simulink library "UndergraduateResearch"  (Simulink 8.1)
settings: Solver=ode45  StartTime=0.0  StopTime=10.0  RelTol=1e-3
undefined symbols (not defined in the file or in its folder): datafiI, datafiQ, i, magnitude
libraries: commchan3 x40, UndergraduateResearch x35, dspxfrm3 x6, dspstat3 x4, dspmtrx3 x4, commseqgen2 x4, dspindex x2, simulink x2, dspbuff3 x1
(part 1 of 2)
settings Model: Creator=dmiralles  LastModifiedBy=dmiralles

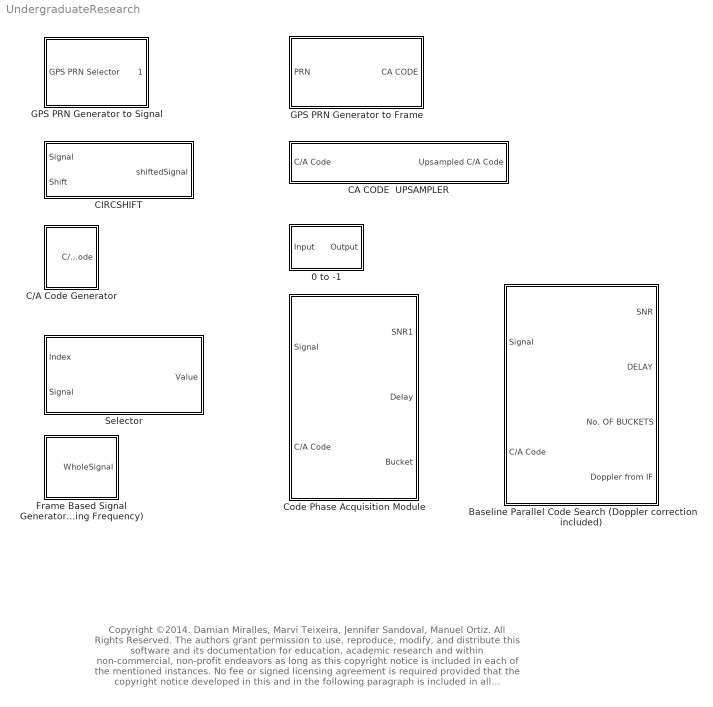
== system UndergraduateResearch ==
  note: Copyright ©2014.  Damian Miralles, Marvi Teixeira, Jennifer Sandoval, Manuel Ortiz. All Rights Reserved.
      | The authors grant permission to use, reproduce, modify, and distribute this software and its documentation for
      | education,  academic research and within non-commercial, non-profit endeavors as long as this copyright notice
      |  is included in each of the mentioned instances. No fee or signed licensing agreement is required provided that
      | the copyright notice developed in this and in the following  paragraph is included in all reproductions,  alterations,
      | and distributions of the software or its  documentation. Contact the authors regarding any commercial licensing needs.
      |
      | THIS EXPERIMENTAL SOFTWARE AND RELATED DOCUMENTATION ARE PROVIDED “AS IS” AND
      |  NO, EXPLICIT OR IMPLICT, CLAIMS REGARDING THEIR ACCURACY OR SUITABILITY ARE MADE.
      | USERS ARE RESPONSIBLE FOR SOFTWARE VALIDATION REGARDING THEIR PARTICULAR
      |  APPLICATION. NO UPDATES WILL BE OFFERED. VERY LIMITED SUPPORT COULD BE PROVIDED,
      |  BUT NOT GUARANTEED, ON A CASE BY CASE BASIS, DEPENDING ON THE AVAILABLE TIME
      |  RESOURCES AT THE TIME OF THE REQUEST.
      | (dmiralles2009@gmail.com,  cc: mteixeir@ieee.org )
  " 0 to -1" : Subsystem  mask(Change 0 to -1){}
      mask help: The blocks performs the conversion of the 0 values to -1. This is used to represent the series as in the polar non-return-to-zero notation which is more easy to handle to perform data analysis.
      mask Help:
      | After code generation, the codes are combined with the navigation data through modulo-2 adders. The exclusive OR operation is used on binary sequences represented by 0’s and 1’s, and its properties are shown in  Table 1.
      | <br>
      | 
      | <table>
      |   <caption>Table 1:Output of the exclusive OR operation</caption>
      |   <tr>
      |     <th>Input</th>
      |     <th>Input</th>
      |     <th>Output</th>
      |   </tr>
      |   <tr>
      |     <td>0</td>
      |     <td>0</td>
      |     <td>0</td>
      |   </tr>
      |   <tr>
      |     <td>0</td>
      |     <td>1</td>
      |     <td>1</td>
      |   </tr>
      |   <tr>
      |     <td>1</td>
      |     <td>0</td>
      |     <td>1</td>
      |   </tr>
      |   <tr>
      |     <td>1</td>
      |     <td>1</td>
      |     <td>0</td>
      |   </tr>
      | </table>
      | 
      | If the binary sequences were represented by the polar non-return-to-zero representation, i.e., 1’s and −1’s, ordinary multiplication could be used instead. The corresponding properties of the multiplication with two binary non-return-to-zero  sequences are shown in Table 2.
      | 
      | <table>
      |   <caption>Table 1:Output of the exclusive OR operation</caption>
      |   <colgroup span="4" class="columns"></colgroup>
      |   <tr>
      |     <th>Input</th>
      |     <th>Input</th>
      |     <th>Output</th>
      |   </tr>
      |   <tr>
      |     <td>-1</td>
      |     <td>-1</td>
      |     <td>1</td>
      |   </tr>
      |   <tr>
      |     <td>-1</td>
      |     <td>1</td>
      |     <td>-1</td>
      |   </tr>
      |   <tr>
      |     <td>1</td>
      |     <td>-1</td>
      |     <td>-1</td>
      |   </tr>
      |   <tr>
      |     <td>1</td>
      |     <td>1</td>
      |     <td>1</td>
      |   </tr>
      | </table>
      | The internals of the block is presented in the illustration below, as can be seen a simple operation of multiplication by 2 and then a sum with -1 will ensure that a binary series will change 0 by -1 and leave the 1 values as such.
  " Selector" : MATLAB Function  TreatAsAtomicUnit=on  mask(Select Element){}
      mask help: The blocks select an element given an index in any vector of matrix input at Signla port. The block have been tested extensively with one column vector or one row vectors.
  Baseline Parallel Code Search (Doppler correction included) : Subsystem  TreatAsAtomicUnit=on  mask{ssize=572880, ifreq=9548000, fs=38192000, satellite=21}
      mask prompts: ssize "Signal Size in Samples"; ifreq "Intermediate Frequency(Hz)"; fs "Sampling Frequency(Hz)"; satellite "Desired Satellite PRN"
      mask help:
      | The block implements the Parallel Code Search Acquisition method of a real time raw GPS signal. The block receives two input parameters, where signal is the raw gps signal and C/A code is the local generated code used as a method of comparison.
      | The block has several parameters to achieve its final functionality, the Signal Size is the size of the signal in samples that would be passed to the code, this value have to be an integer multiple of (sampling frequency/1000).
      | The intermediate frequency, expressed in Hertz , is the frequency to which the carrier frequency is shifted as an intermediate step in transmission or reception.
      | The sampling frequency defines the number of samples per unit of time (usually seconds) taken from a continuous signal to make a discrete signal.
      | The Desireed Satellite parameter defines the satellite that the user whcih to target in the simulation process if it is expected to be on the raw signal.
  C/A Code Generator : Subsystem  mask{fs=4092000, sat=1}
      mask prompts: fs "Sampling Frequency (Hz)"; sat "Desired Satellite PRN"
  CA CODE  UPSAMPLER : Subsystem  TreatAsAtomicUnit=on  mask(C/A Code Upsampler){fs=4092000}
      mask prompts: fs "Desired Sampling Frequency (Hz)"
      mask help:
      | The block performs an upsampling to the input signal by intrpolating the samples tp the desired sampling frequency. Once it's specified the desired sampling frequency the block would interpolate the input samples untill the new desired sampling frequency is desired.
      | The block is dependable on receiving an input signal of 1023 samples for the desired GPS, and the output signal would have a length of fs/1000 samples corresponding to the interpolated signal.
  CIRCSHIFT : MATLAB Function  TreatAsAtomicUnit=on  mask(CircularShift){}
      mask help: The block performs a circular shift of the Signal by the amount specified by Shift, the block is equivalent to the "circshift" function of MATLAB
  Code Phase Acquisition Module : Subsystem  TreatAsAtomicUnit=on  mask{fs=4092000}
      mask prompts: fs "Sampling Frequency"
  Frame Based Signal Generator (Any Sampling Frequency) : Subsystem  mask{satellites=[1 2 3 4 5 6 7 8 9], d1=378, interference=[10 20 30 40 50 60 70 80 90], gain=[0.1 0.2 0.3 0.4 0.5 0.6 0.7 0.8 0.9], snr=-20, fs=4092000}
      mask prompts: satellites "List of Satellites(1:9)"; d1 "Desired Satellite Delay"; interference "Interference Delay Vector(1:9) *First entry is for multipath delay"; gain "Interference Gain Vector(1:9) *First entry is for multipath attenuation"; snr "SNR (dB) for AWGN"; fs "Desired Sampling Frequency(Hz)"
  GPS PRN Generator to Frame : Subsystem  TreatAsAtomicUnit=on  mask(GPS PRN Generator Frame Based){}
      mask help:
      | The block generates the 1023 bits long C/A sequence. The input to the block is a constant value that specifies the desired PRN code. Take into consideration that the legal input values are between 1 and 37.The block generates a frame based output of 1023 samples not dependable on the simulation time.
      | It is recommended to set the simulation parameters to execute a single step simulation in order to generate the desired code.
  GPS PRN Generator to Signal : Subsystem  mask(GPS PRN Generator Continous){}
      mask help: The block generates the 1023 bits long C/A sequence. The input to the block is a constant value that specifies the desired PRN code. Take into consideration that the legal input values are between 1 and 37. The block is of continuous heritage so the blocks function with the simulation time accordinly.The blocks needs n step size to generate the n long code, so for GPS purpose set the simulation parameters to run 1023 steps per code.

== system UndergraduateResearch/ 0 to -1 ==
  Input : Inport
  " " : Constant  Value=2
  "   " : Product  RndMeth=Zero
  "     " : Constant  Value=-1
  Sum : Sum  Inputs=|++
  Output : Outport
  wires:
  " "/1 -> "   "/2
  Sum/1 -> Output/1
  Input/1 -> "   "/1
  "     "/1 -> Sum/2
  "   "/1 -> Sum/1

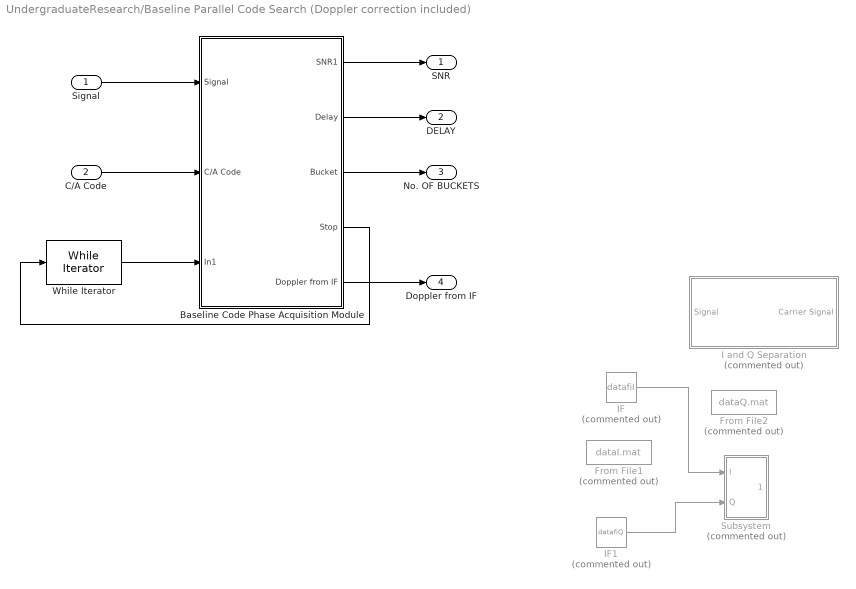
== system UndergraduateResearch/Baseline Parallel Code Search (Doppler correction included) ==
  Signal : Inport
  C/A Code : Inport  Port=2
  Baseline Code Phase Acquisition Module : Subsystem  TreatAsAtomicUnit=on  mask{fs=fs}
      mask prompts: fs "Sampling Frequency"
  From File1 : FromFile  Commented=on  FileName=dataI.mat  SampleTime=0
  From File2 : FromFile  Commented=on  FileName=dataQ.mat  SampleTime=0
  I and Q Separation : Subsystem  Commented=on  mask{ifreq=ifreq, ss=ssize, fs=fs}
      mask prompts: ifreq "Intermediate Frequency (Hz)"; ss "Signal Size"; fs "Sampling Frequency (Hz)"
  IF : Constant  Commented=on  Value=datafiI
  IF1 : Constant  Commented=on  Value=datafiQ
  Subsystem : Subsystem  Commented=on
  While Iterator : WhileIterator  MaxIters=21  WhileBlockType=do-while  ResetStates=reset  ShowIterationPort=on
  SNR : Outport
  DELAY : Outport  Port=2
  No. OF BUCKETS : Outport  Port=3
  Doppler from IF : Outport  Port=4
  wires:
  Signal/1 -> Baseline Code Phase Acquisition Module/1(Signal)
  C/A Code/1 -> Baseline Code Phase Acquisition Module/2(C/A Code)
  IF1/1 -> Subsystem/2(Q)
  IF/1 -> Subsystem/1(I)
  Baseline Code Phase Acquisition Module/5(Doppler from IF) -> Doppler from IF/1
  Baseline Code Phase Acquisition Module/4(Stop) -> While Iterator/1
  While Iterator/1 -> Baseline Code Phase Acquisition Module/3(In1)
  Baseline Code Phase Acquisition Module/3(Bucket) -> No. OF BUCKETS/1
  Baseline Code Phase Acquisition Module/2(Delay) -> DELAY/1
  Baseline Code Phase Acquisition Module/1(SNR1) -> SNR/1

== system UndergraduateResearch/C/A Code Generator ==
  CA CODE  UPSAMPLER1 : UndergraduateResearch/CA CODE  UPSAMPLER  fs=fs
  Constant : Constant  Value=sat
  GPS PRN Generator to Frame1 : UndergraduateResearch/GPS PRN Generator to Frame
  C/A Code : Outport
  wires:
  Constant/1 -> GPS PRN Generator to Frame1/1
  CA CODE  UPSAMPLER1/1 -> C/A Code/1
  GPS PRN Generator to Frame1/1 -> CA CODE  UPSAMPLER1/1

== system UndergraduateResearch/CA CODE  UPSAMPLER ==
  C/A Code : Inport
  " Selector" : MATLAB Function  TreatAsAtomicUnit=on
  Buffering Line : dspbuff3/Delay Line  siz=floor(fs/1000)  ic=0  directfeed=on  enable_output=off  hold_output=off  TreatMby1Signals=One channel
  Ceiling : Fcn  Expr=ceil(u)
  Iterator : ForIterator  ResetStates=reset  IterationLimit=floor(fs/1000)
  Multiplier : Product
  Sampling Frequency : Constant  Value=1023000/fs
  Signal Size : Constant  Value=1023
  Switch : Switch  Criteria=u2 > Threshold  Threshold=1023
  Upsampled C/A Code : Outport
  wires:
  Sampling Frequency/1 -> Multiplier/2
  Multiplier/1 -> Ceiling/1
  Signal Size/1 -> Switch/1
  Iterator/1 -> Multiplier/1
  Ceiling/1 -> Switch/3, Switch/2
  Switch/1 -> " Selector"/1(Index)
  C/A Code/1 -> " Selector"/2(Signal)
  " Selector"/1(Value) -> Buffering Line/1
  Buffering Line/1 -> Upsampled C/A Code/1

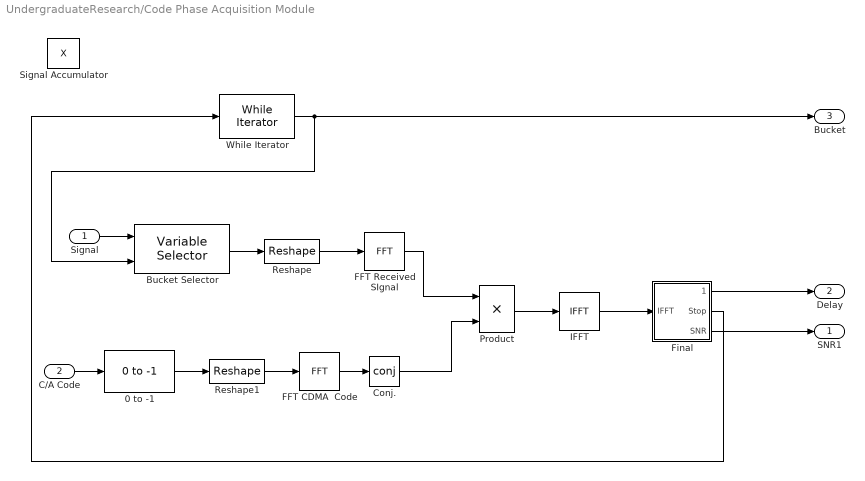
== system UndergraduateResearch/Code Phase Acquisition Module ==
  Signal : Inport
  C/A Code : Inport  Port=2
  " 0 to -1" : UndergraduateResearch/ 0 to -1
  Bucket Selector : dspindex/Variable Selector  NumInputs=1  rowsOrCols=Rows  IdxMode=Variable  Elements=[1 3]  ZerOneIdxMode=One-based  errmode=Clip Index  FillMode=on  FillValues=0
  Conj. : Math  Operator=conj  SaturateOnIntegerOverflow=on
  FFT CDMA  Code : dspxfrm3/FFT  CompMethod=Table lookup  TableOpt=NEW  TableOptActive=Speed  BitRevOrder=off  InheritFFTLength=on  FFTLength=1024  RowConvenienceOn=on  FFTImplementation=FFTW  SkipNorm=off  firstCoeffDataTypeStr=Inherit: Same word length as input  firstCoeffLastDataTypeStr=Inherit: Same word length as input  outputMin=[]  outputMax=[]  roundingMode=Floor  overflowMode=off
  FFT Received SIgnal : dspxfrm3/FFT  CompMethod=Table lookup  TableOpt=NEW  TableOptActive=Speed  BitRevOrder=off  InheritFFTLength=on  FFTLength=1024  RowConvenienceOn=on  FFTImplementation=FFTW  SkipNorm=off  firstCoeffDataTypeStr=Inherit: Same word length as input  firstCoeffLastDataTypeStr=Inherit: Same word length as input  outputMin=[]  outputMax=[]  roundingMode=Floor  overflowMode=off
  Final : Subsystem
      mask help:
      | The Final block receives an IFFT and returns if the SNR passed the threshhold
      | and also outputs the SNR and the delay. It uses a variable to accumulate the signal
      | adds it to IFFT and stores it. It detects the maximum value in the signal with the index and assings a 0
      | to remove the peak to be able to calculate the mean and obtain the SNR.
  IFFT : dspxfrm3/IFFT  CompMethod=Table lookup  TableOpt=NEW  TableOptActive=Speed  BitRevOrder=off  cs_in=off  SkipNorm=off  InheritFFTLength=on  FFTLength=1024  mode=Complex  outSamplingMode=Sample based  RowConvenienceOn=on  FFTImplementation=FFTW  firstCoeffDataTypeStr=Inherit: Same word length as input  firstCoeffLastDataTypeStr=Inherit: Same word length as input  outputMin=[]  outputMax=[]  roundingMode=Floor  overflowMode=off
  Product : Product  RndMeth=Zero
  Reshape : Reshape  OutputDimensions=[1023,40]
  Reshape1 : Reshape  OutputDimensions=[1023,40]
  Signal Accumulator : DataStoreMemory  DataStoreName=X  ReadBeforeWriteMsg=warning  WriteAfterWriteMsg=warning  WriteAfterReadMsg=warning  InitialValue=zeros(1,floor(fs/1000))  VectorParams1D=off
  While Iterator : WhileIterator  MaxIters=20  WhileBlockType=do-while  ShowIterationPort=on  OutputDataType=double
  SNR1 : Outport
  Delay : Outport  Port=2
  Bucket : Outport  Port=3
  wires:
  FFT CDMA  Code/1 -> Conj./1
  FFT Received SIgnal/1 -> Product/1
  Conj./1 -> Product/2
  Product/1 -> IFFT/1
  Signal/1 -> Bucket Selector/1
  While Iterator/1 -> Bucket Selector/2, Bucket/1
  IFFT/1 -> Final/1(IFFT)
  Final/1(Delay) -> Delay/1
  Final/3("SNR ") -> SNR1/1
  Final/2(Stop) -> While Iterator/1
  C/A Code/1 -> " 0 to -1"/1
  Reshape/1 -> FFT Received SIgnal/1
  Bucket Selector/1 -> Reshape/1
  Reshape1/1 -> FFT CDMA  Code/1
  " 0 to -1"/1 -> Reshape1/1

== system UndergraduateResearch/Frame Based Signal Generator (Any Sampling Frequency) ==
  BasebandSignal : Subsystem
  Noise Addition : Subsystem
  Reshape : Reshape  OutputDimensionality=Customize  OutputDimensions=[floor(fs/1000),40]
  Transpose : dspmtrx3/Transpose  Hermitian=off  overflowFlag=off
  WholeSignal : Outport
  wires:
  Reshape/1 -> Transpose/1
  Transpose/1 -> WholeSignal/1
  Noise Addition/1(Out1) -> Reshape/1
  BasebandSignal/1(Signal) -> Noise Addition/1(In1)

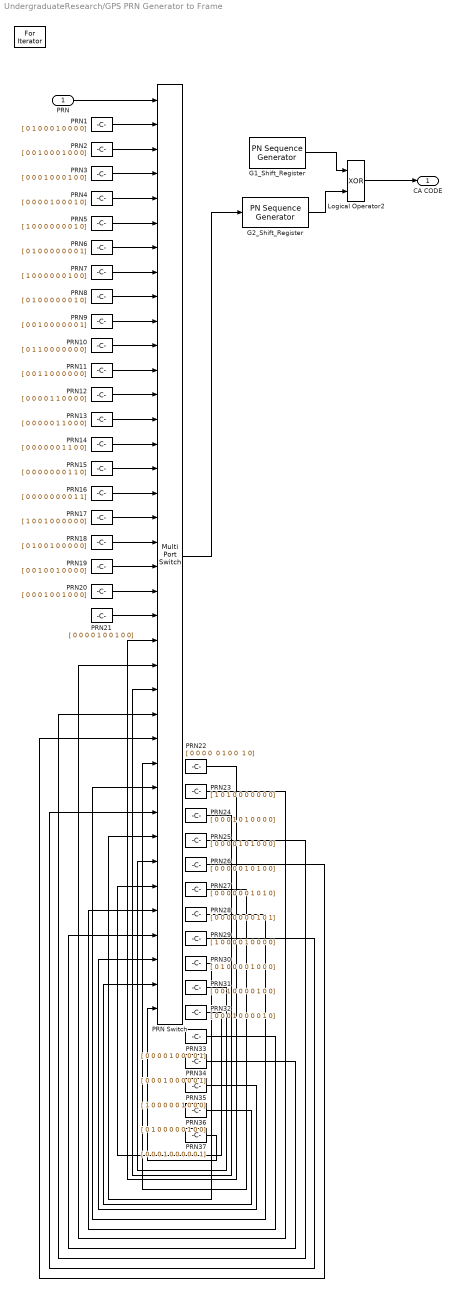
== system UndergraduateResearch/GPS PRN Generator to Frame ==
  PRN : Inport
  " " : ForIterator  IterationLimit=1023
  G1_Shift_Register : commseqgen2/PN Sequence Generator  poly=[10 7 0]  ini_sta=[1 1 1 1 1 1 1 1 1 1]  outBitMaskSource=Dialog parameter  shift=[0 0 0 0 0 0 0 0 0 1]  outVarSiz=off  maxOutSizeMode=Dialog parameter  maxOutSize=[10 1]  Ts=-1  frameBased=on  sampPerFrame=1023  reset=off  bitPackedOutputs=off  outDataType=double  numPackedBits=8  bitPackDataSigned=off  bitPackedOutDType=double
  G2_Shift_Register : commseqgen2/PN Sequence Generator  poly=[10 8 7 4 2 1 0]  ini_sta=[1 1 1 1 1 1 1 1 1 1]  outBitMaskSource=Input port  shift=[ 0 1 0 0 0 1 0 0 0 0]  outVarSiz=off  maxOutSizeMode=Dialog parameter  maxOutSize=[10 1]  Ts=-1  frameBased=on  sampPerFrame=1023  reset=off  bitPackedOutputs=off  outDataType=double  numPackedBits=8  bitPackDataSigned=off  bitPackedOutDType=double
  Logical Operator2 : Logic  Operator=XOR  AllPortsSameDT=off  OutDataTypeStr=boolean
  PRN Switch : MultiPortSwitch  Inputs=37
  PRN1 : Constant  Value=[ 0 1 0 0 0 1 0 0 0 0]
  PRN10 : Constant  Value=[ 0 1 1 0 0 0 0 0 0 0]
  PRN11 : Constant  Value=[ 0 0 1 1 0 0 0 0 0 0]
  PRN12 : Constant  Value=[ 0 0 0 0 1 1 0 0 0 0]
  PRN13 : Constant  Value=[ 0 0 0 0 0 1 1 0 0 0]
  PRN14 : Constant  Value=[ 0 0 0 0 0 0 1 1 0 0]
  PRN15 : Constant  Value=[ 0 0 0 0 0 0 0 1 1 0]
  PRN16 : Constant  Value=[ 0 0 0 0 0 0 0 0 1 1]
  PRN17 : Constant  Value=[ 1 0 0 1 0 0 0 0 0 0]
  PRN18 : Constant  Value=[ 0 1 0 0 1 0 0 0 0 0]
  PRN19 : Constant  Value=[ 0 0 1 0 0 1 0 0 0 0]
  PRN2 : Constant  Value=[ 0 0 1 0 0 0 1 0 0 0]
  PRN20 : Constant  Value=[ 0 0 0 1 0 0 1 0 0 0]
  PRN21 : Constant  Value=[ 0 0 0 0 1 0 0 1 0 0]
  PRN22 : Constant  Value="[ 0 0 0 0  0 1 0 0  1 0]"
  PRN23 : Constant  Value=[ 1 0 1 0 0 0 0 0 0 0]
  PRN24 : Constant  Value=[ 0 0 0 1 0 1 0 0 0 0]
  PRN25 : Constant  Value=[ 0 0 0 0 1 0 1 0 0 0]
  PRN26 : Constant  Value=[ 0 0 0 0 0 1 0 1 0 0]
  PRN27 : Constant  Value=[ 0 0 0 0 0 0 1 0 1 0]
  PRN28 : Constant  Value=[ 0 0 0 0 0 0 0 1 0 1]
  PRN29 : Constant  Value=[ 1 0 0 0 0 1 0 0 0 0]
  PRN3 : Constant  Value=[ 0 0 0 1 0 0 0 1 0 0]
  PRN30 : Constant  Value=[ 0 1 0 0 0 0 1 0 0 0]
  PRN31 : Constant  Value=[ 0 0 1 0 0 0 0 1 0 0]
  PRN32 : Constant  Value=[ 0 0 0 1 0 0 0 0 1 0]
  PRN33 : Constant  Value=[ 0 0 0 0 1 0 0 0 0 1]
  PRN34 : Constant  Value=[ 0 0 0 1 0 0 0 0 0 1]
  PRN35 : Constant  Value=[ 1 0 0 0 0 0 1 0 0 0]
  PRN36 : Constant  Value=[ 0 1 0 0 0 0 0 1 0 0]
  PRN37 : Constant  Value=[ 0 0 0 1 0 0 0 0 0 1]
  PRN4 : Constant  Value=[ 0 0 0 0 1 0 0 0 1 0]
  PRN5 : Constant  Value=[ 1 0 0 0 0 0 0 0 1 0]
  PRN6 : Constant  Value=[ 0 1 0 0 0 0 0 0 0 1]
  PRN7 : Constant  Value=[ 1 0 0 0 0 0 0 1 0 0]
  PRN8 : Constant  Value=[ 0 1 0 0 0 0 0 0 1 0]
  PRN9 : Constant  Value=[ 0 0 1 0 0 0 0 0 0 1]
  CA CODE : Outport
  wires:
  PRN24/1 -> PRN Switch/25
  PRN22/1 -> PRN Switch/23
  PRN20/1 -> PRN Switch/21
  PRN27/1 -> PRN Switch/28
  PRN11/1 -> PRN Switch/12
  PRN36/1 -> PRN Switch/37
  PRN13/1 -> PRN Switch/14
  PRN12/1 -> PRN Switch/13
  PRN8/1 -> PRN Switch/9
  PRN25/1 -> PRN Switch/26
  PRN29/1 -> PRN Switch/30
  G2_Shift_Register/1 -> Logical Operator2/2
  PRN7/1 -> PRN Switch/8
  PRN26/1 -> PRN Switch/27
  PRN5/1 -> PRN Switch/6
  PRN30/1 -> PRN Switch/31
  PRN19/1 -> PRN Switch/20
  PRN18/1 -> PRN Switch/19
  PRN35/1 -> PRN Switch/36
  PRN33/1 -> PRN Switch/34
  PRN9/1 -> PRN Switch/10
  PRN1/1 -> PRN Switch/2
  PRN17/1 -> PRN Switch/18
  PRN23/1 -> PRN Switch/24
  PRN3/1 -> PRN Switch/4
  PRN37/1 -> PRN Switch/38
  PRN2/1 -> PRN Switch/3
  PRN21/1 -> PRN Switch/22
  PRN4/1 -> PRN Switch/5
  PRN10/1 -> PRN Switch/11
  PRN6/1 -> PRN Switch/7
  PRN32/1 -> PRN Switch/33
  PRN31/1 -> PRN Switch/32
  G1_Shift_Register/1 -> Logical Operator2/1
  PRN15/1 -> PRN Switch/16
  PRN Switch/1 -> G2_Shift_Register/1
  PRN16/1 -> PRN Switch/17
  PRN14/1 -> PRN Switch/15
  PRN/1 -> PRN Switch/1
  PRN34/1 -> PRN Switch/35
  PRN28/1 -> PRN Switch/29
  Logical Operator2/1 -> CA CODE/1

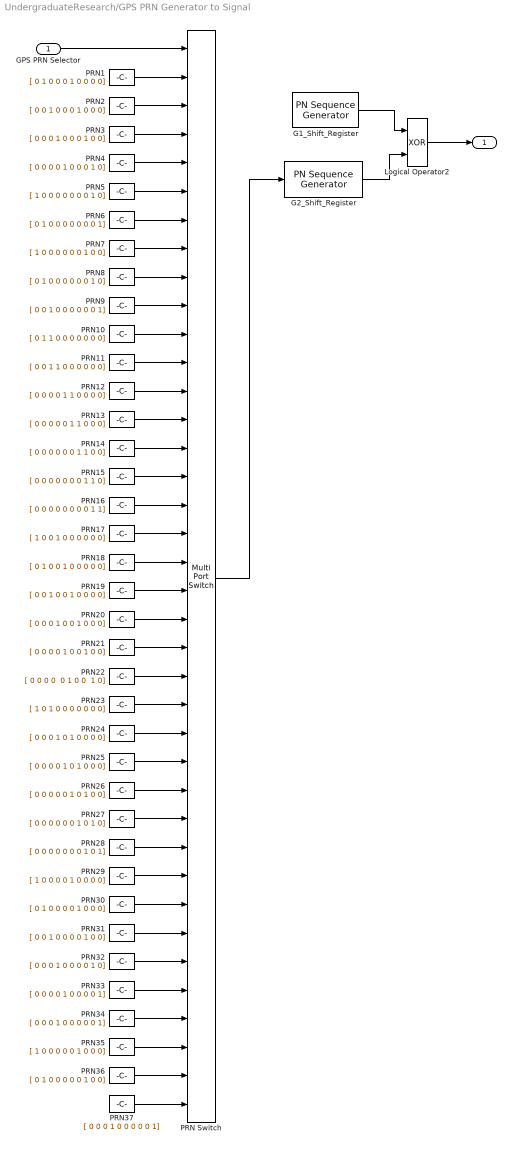
== system UndergraduateResearch/GPS PRN Generator to Signal ==
  GPS PRN Selector : Inport
  G1_Shift_Register : commseqgen2/PN Sequence Generator  poly=[10 7 0]  ini_sta=[1 1 1 1 1 1 1 1 1 1]  outBitMaskSource=Dialog parameter  shift=[0 0 0 0 0 0 0 0 0 1]  outVarSiz=off  maxOutSizeMode=Dialog parameter  maxOutSize=[10 1]  Ts=1  frameBased=off  sampPerFrame=1  reset=off  bitPackedOutputs=off  outDataType=double  numPackedBits=8  bitPackDataSigned=off  bitPackedOutDType=double
  G2_Shift_Register : commseqgen2/PN Sequence Generator  poly=[10 8 7 4 2 1 0]  ini_sta=[1 1 1 1 1 1 1 1 1 1]  outBitMaskSource=Input port  shift=[ 0 1 0 0 0 1 0 0 0 0]  outVarSiz=off  maxOutSizeMode=Dialog parameter  maxOutSize=[10 1]  Ts=1  frameBased=off  sampPerFrame=1  reset=off  bitPackedOutputs=off  outDataType=double  numPackedBits=8  bitPackDataSigned=off  bitPackedOutDType=double
  Logical Operator2 : Logic  Operator=XOR  AllPortsSameDT=off  OutDataTypeStr=boolean
  PRN Switch : MultiPortSwitch  Inputs=37
  PRN1 : Constant  Value=[ 0 1 0 0 0 1 0 0 0 0]
  PRN10 : Constant  Value=[ 0 1 1 0 0 0 0 0 0 0]
  PRN11 : Constant  Value=[ 0 0 1 1 0 0 0 0 0 0]
  PRN12 : Constant  Value=[ 0 0 0 0 1 1 0 0 0 0]
  PRN13 : Constant  Value=[ 0 0 0 0 0 1 1 0 0 0]
  PRN14 : Constant  Value=[ 0 0 0 0 0 0 1 1 0 0]
  PRN15 : Constant  Value=[ 0 0 0 0 0 0 0 1 1 0]
  PRN16 : Constant  Value=[ 0 0 0 0 0 0 0 0 1 1]
  PRN17 : Constant  Value=[ 1 0 0 1 0 0 0 0 0 0]
  PRN18 : Constant  Value=[ 0 1 0 0 1 0 0 0 0 0]
  PRN19 : Constant  Value=[ 0 0 1 0 0 1 0 0 0 0]
  PRN2 : Constant  Value=[ 0 0 1 0 0 0 1 0 0 0]
  PRN20 : Constant  Value=[ 0 0 0 1 0 0 1 0 0 0]
  PRN21 : Constant  Value=[ 0 0 0 0 1 0 0 1 0 0]
  PRN22 : Constant  Value="[ 0 0 0 0  0 1 0 0  1 0]"
  PRN23 : Constant  Value=[ 1 0 1 0 0 0 0 0 0 0]
  PRN24 : Constant  Value=[ 0 0 0 1 0 1 0 0 0 0]
  PRN25 : Constant  Value=[ 0 0 0 0 1 0 1 0 0 0]
  PRN26 : Constant  Value=[ 0 0 0 0 0 1 0 1 0 0]
  PRN27 : Constant  Value=[ 0 0 0 0 0 0 1 0 1 0]
  PRN28 : Constant  Value=[ 0 0 0 0 0 0 0 1 0 1]
  PRN29 : Constant  Value=[ 1 0 0 0 0 1 0 0 0 0]
  PRN3 : Constant  Value=[ 0 0 0 1 0 0 0 1 0 0]
  PRN30 : Constant  Value=[ 0 1 0 0 0 0 1 0 0 0]
  PRN31 : Constant  Value=[ 0 0 1 0 0 0 0 1 0 0]
  PRN32 : Constant  Value=[ 0 0 0 1 0 0 0 0 1 0]
  PRN33 : Constant  Value=[ 0 0 0 0 1 0 0 0 0 1]
  PRN34 : Constant  Value=[ 0 0 0 1 0 0 0 0 0 1]
  PRN35 : Constant  Value=[ 1 0 0 0 0 0 1 0 0 0]
  PRN36 : Constant  Value=[ 0 1 0 0 0 0 0 1 0 0]
  PRN37 : Constant  Value=[ 0 0 0 1 0 0 0 0 0 1]
  PRN4 : Constant  Value=[ 0 0 0 0 1 0 0 0 1 0]
  PRN5 : Constant  Value=[ 1 0 0 0 0 0 0 0 1 0]
  PRN6 : Constant  Value=[ 0 1 0 0 0 0 0 0 0 1]
  PRN7 : Constant  Value=[ 1 0 0 0 0 0 0 1 0 0]
  PRN8 : Constant  Value=[ 0 1 0 0 0 0 0 0 1 0]
  PRN9 : Constant  Value=[ 0 0 1 0 0 0 0 0 0 1]
  " " : Outport
  wires:
  PRN23/1 -> PRN Switch/24
  PRN24/1 -> PRN Switch/25
  PRN25/1 -> PRN Switch/26
  PRN29/1 -> PRN Switch/30
  PRN26/1 -> PRN Switch/27
  PRN27/1 -> PRN Switch/28
  PRN28/1 -> PRN Switch/29
  PRN31/1 -> PRN Switch/32
  PRN34/1 -> PRN Switch/35
  PRN37/1 -> PRN Switch/38
  PRN30/1 -> PRN Switch/31
  PRN32/1 -> PRN Switch/33
  PRN35/1 -> PRN Switch/36
  PRN33/1 -> PRN Switch/34
  PRN36/1 -> PRN Switch/37
  PRN2/1 -> PRN Switch/3
  GPS PRN Selector/1 -> PRN Switch/1
  PRN7/1 -> PRN Switch/8
  PRN8/1 -> PRN Switch/9
  PRN9/1 -> PRN Switch/10
  PRN10/1 -> PRN Switch/11
  PRN12/1 -> PRN Switch/13
  PRN11/1 -> PRN Switch/12
  PRN13/1 -> PRN Switch/14
  PRN14/1 -> PRN Switch/15
  PRN15/1 -> PRN Switch/16
  PRN16/1 -> PRN Switch/17
  PRN18/1 -> PRN Switch/19
  PRN19/1 -> PRN Switch/20
  PRN20/1 -> PRN Switch/21
  PRN21/1 -> PRN Switch/22
  PRN22/1 -> PRN Switch/23
  G2_Shift_Register/1 -> Logical Operator2/2
  PRN Switch/1 -> G2_Shift_Register/1
  PRN1/1 -> PRN Switch/2
  PRN6/1 -> PRN Switch/7
  PRN4/1 -> PRN Switch/5
  PRN5/1 -> PRN Switch/6
  PRN3/1 -> PRN Switch/4
  PRN17/1 -> PRN Switch/18
  G1_Shift_Register/1 -> Logical Operator2/1
  Logical Operator2/1 -> " "/1

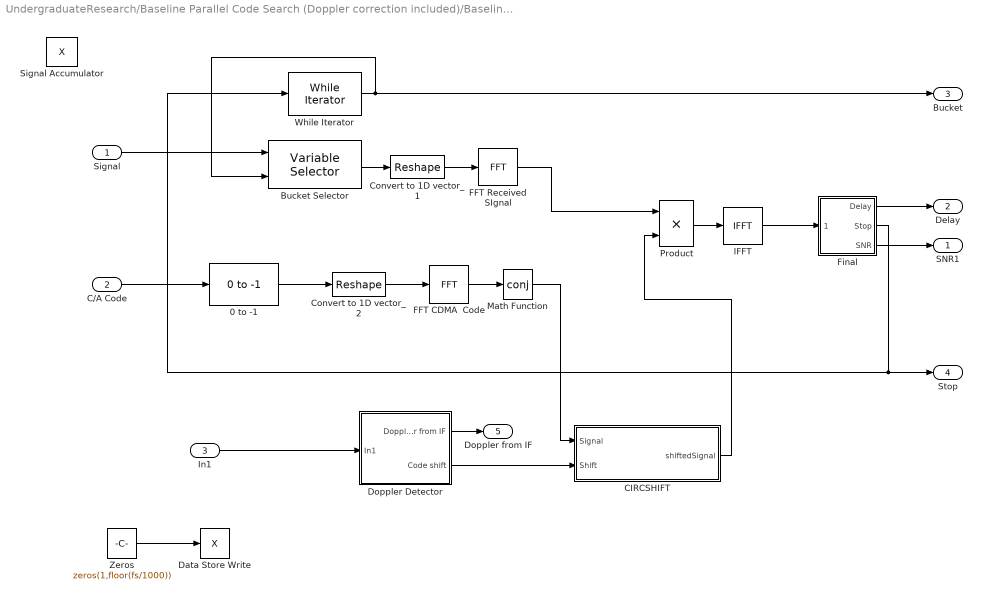
== system UndergraduateResearch/Baseline Parallel Code Search (Doppler correction included)/Baseline Code Phase Acquisition Module ==
  Signal : Inport
  C/A Code : Inport  Port=2
  In1 : Inport  Port=3
  " 0 to -1" : UndergraduateResearch/ 0 to -1
  Bucket Selector : dspindex/Variable Selector  NumInputs=1  rowsOrCols=Rows  IdxMode=Variable  Elements=[1 3]  ZerOneIdxMode=One-based  errmode=Clip Index  FillMode=off  FillValues=0
  CIRCSHIFT : MATLAB Function  TreatAsAtomicUnit=on  mask(CircularShift){}
      mask help: The block performs a circular shift of the Signal by the amount specified by Shift, the block is equivalent to the "circshift" function of MATLAB
  Convert to 1D vector_1 : Reshape  OutputDimensions=[1023,40]
  Convert to 1D vector_2 : Reshape  OutputDimensions=[1023,40]
  Data Store Write : DataStoreWrite  DataStoreName=X
  Doppler Detector : Subsystem
  FFT CDMA  Code : dspxfrm3/FFT  CompMethod=Table lookup  TableOpt=NEW  TableOptActive=Speed  BitRevOrder=off  InheritFFTLength=on  FFTLength=1024  RowConvenienceOn=on  FFTImplementation=FFTW  SkipNorm=off  firstCoeffDataTypeStr=Inherit: Same word length as input  firstCoeffLastDataTypeStr=Inherit: Same word length as input  outputMin=[]  outputMax=[]  roundingMode=Floor  overflowMode=off
  FFT Received SIgnal : dspxfrm3/FFT  CompMethod=Table lookup  TableOpt=NEW  TableOptActive=Speed  BitRevOrder=off  InheritFFTLength=on  FFTLength=1024  RowConvenienceOn=on  FFTImplementation=FFTW  SkipNorm=off  firstCoeffDataTypeStr=Inherit: Same word length as input  firstCoeffLastDataTypeStr=Inherit: Same word length as input  outputMin=[]  outputMax=[]  roundingMode=Floor  overflowMode=off
  Final : Subsystem
      mask help: The Final block receives an IFFT and returns if the SNR passed the threshhold and also outputs the SNR and the delay. It uses a variable to accumulate the signal adds it to IFFT and stores it. It detects the maximum value in the signal with the index and assings a 0 to remove the peak to be able to calculate the mean and obtain the SNR.
  IFFT : dspxfrm3/IFFT  CompMethod=Table lookup  TableOpt=NEW  TableOptActive=Speed  BitRevOrder=off  cs_in=off  SkipNorm=on  InheritFFTLength=on  FFTLength=1024  mode=Complex  outSamplingMode=Sample based  RowConvenienceOn=on  FFTImplementation=FFTW  firstCoeffDataTypeStr=Inherit: Same word length as input  firstCoeffLastDataTypeStr=Inherit: Same word length as input  outputMin=[]  outputMax=[]  roundingMode=Floor  overflowMode=off
  Math Function : Math  Operator=conj  SaturateOnIntegerOverflow=on
  Product : Product  RndMeth=Zero
  Signal Accumulator : DataStoreMemory  DataStoreName=X  ReadBeforeWriteMsg=warning  WriteAfterWriteMsg=warning  WriteAfterReadMsg=warning  InitialValue=zeros(1,floor(fs/1000))  VectorParams1D=off
  While Iterator : WhileIterator  MaxIters=10  WhileBlockType=do-while  ResetStates=reset  ShowIterationPort=on  OutputDataType=double
  Zeros : Constant  Value=zeros(1,floor(fs/1000))
  SNR1 : Outport
  Delay : Outport  Port=2
  Bucket : Outport  Port=3
  Stop : Outport  Port=4
  Doppler from IF : Outport  Port=5
  wires:
  Zeros/1 -> Data Store Write/1
  Convert to 1D vector_1/1 -> FFT Received SIgnal/1
  Bucket Selector/1 -> Convert to 1D vector_1/1
  Doppler Detector/2(Code shift) -> CIRCSHIFT/2(Shift)
  CIRCSHIFT/1(shiftedSignal) -> Product/2
  Math Function/1 -> CIRCSHIFT/1(Signal)
  In1/1 -> Doppler Detector/1(In1)
  Doppler Detector/1(Doppler from IF) -> Doppler from IF/1
  " 0 to -1"/1 -> Convert to 1D vector_2/1
  C/A Code/1 -> " 0 to -1"/1
  Convert to 1D vector_2/1 -> FFT CDMA  Code/1
  Final/2(Stop) -> Stop/1, While Iterator/1
  Final/3("SNR ") -> SNR1/1
  Final/1(Delay) -> Delay/1
  IFFT/1 -> Final/1(" ")
  While Iterator/1 -> Bucket Selector/2, Bucket/1
  Signal/1 -> Bucket Selector/1
  Product/1 -> IFFT/1
  FFT Received SIgnal/1 -> Product/1
  FFT CDMA  Code/1 -> Math Function/1

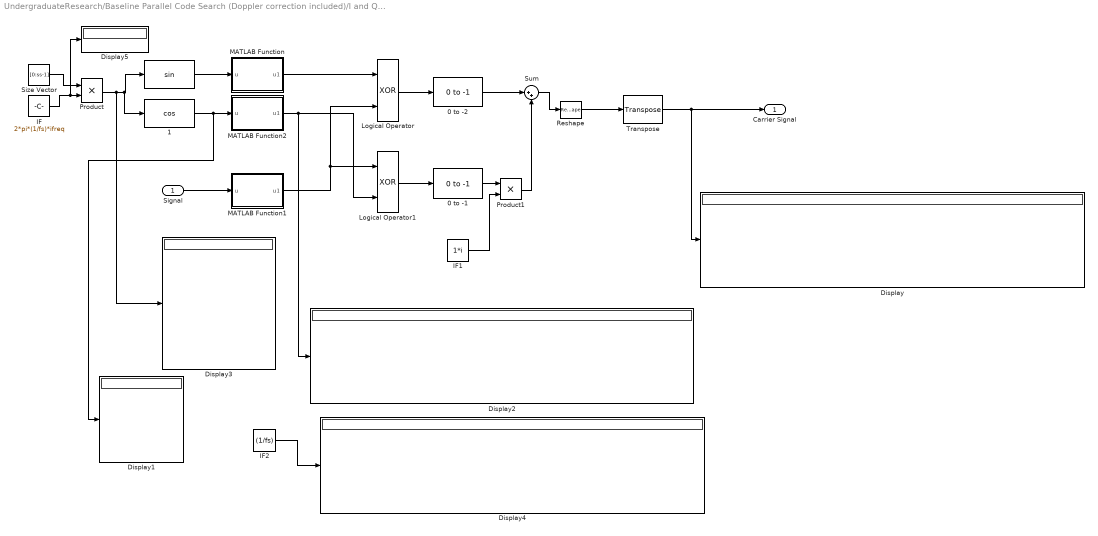
== system UndergraduateResearch/Baseline Parallel Code Search (Doppler correction included)/I and Q Separation ==
  Signal : Inport
  " " : Trigonometry
  " 0 to -1" : UndergraduateResearch/ 0 to -1
  " 0 to -2" : UndergraduateResearch/ 0 to -1
  " 1" : Trigonometry  Operator=cos
  Display{,1..5} (6 alike) : Display
      Display4 settings: Format=long_e
  IF : Constant  Value=2*pi*(1/fs)*ifreq
  IF1 : Constant  Value=1*i
  IF2 : Constant  Value=(1/fs)
  Logical Operator : Logic  Operator=XOR  AllPortsSameDT=off  OutDataTypeStr=boolean
  Logical Operator1 : Logic  Operator=XOR  AllPortsSameDT=off  OutDataTypeStr=boolean
  MATLAB Function : MATLAB Function  TreatAsAtomicUnit=on
  MATLAB Function1 : MATLAB Function  TreatAsAtomicUnit=on
  MATLAB Function2 : MATLAB Function  TreatAsAtomicUnit=on
  Product : Product
  Product1 : Product
  Reshape : Reshape  OutputDimensionality=Customize  OutputDimensions=[38192,15]
  Size Vector : Constant  Value=[0:ss-1]
  Sum : Sum  Inputs=|++
  Transpose : dspmtrx3/Transpose  Hermitian=off  overflowFlag=off
  Carrier Signal : Outport
  wires:
  IF2/1 -> Display4/1
  Sum/1 -> Reshape/1
  IF1/1 -> Product1/2
  Product1/1 -> Sum/2
  " 0 to -1"/1 -> Product1/1
  " 0 to -2"/1 -> Sum/1
  Logical Operator/1 -> " 0 to -2"/1
  Logical Operator1/1 -> " 0 to -1"/1
  MATLAB Function2/1(u1) -> Logical Operator1/2, Display2/1
  " 1"/1 -> MATLAB Function2/1(u), Display1/1
  Signal/1 -> MATLAB Function1/1(u)
  MATLAB Function1/1(u1) -> Logical Operator/2, Logical Operator1/1
  MATLAB Function/1(u1) -> Logical Operator/1
  " "/1 -> MATLAB Function/1(u)
  Transpose/1 -> Carrier Signal/1, Display/1
  Reshape/1 -> Transpose/1
  IF/1 -> Product/2, Display5/1
  Product/1 -> " "/1, " 1"/1, Display3/1
  Size Vector/1 -> Product/1

== system UndergraduateResearch/Baseline Parallel Code Search (Doppler correction included)/Subsystem ==
  I : Inport
  Q : Inport  Port=2
  " 0 to -1" : UndergraduateResearch/ 0 to -1
  " 0 to -2" : UndergraduateResearch/ 0 to -1
  IF1 : Constant  Value=1*i
  Product1 : Product
  Reshape1 : Reshape  OutputDimensionality=Customize  OutputDimensions=[38192,15]
  Sum : Sum  Inputs=|++
  Transpose1 : dspmtrx3/Transpose  Hermitian=off  overflowFlag=off
  Wholesignal : Outport
  wires:
  IF1/1 -> Product1/2
  " 0 to -1"/1 -> Product1/1
  Q/1 -> " 0 to -1"/1
  I/1 -> " 0 to -2"/1
  Product1/1 -> Sum/2
  Sum/1 -> Reshape1/1
  Transpose1/1 -> Wholesignal/1
  Reshape1/1 -> Transpose1/1
  " 0 to -2"/1 -> Sum/1

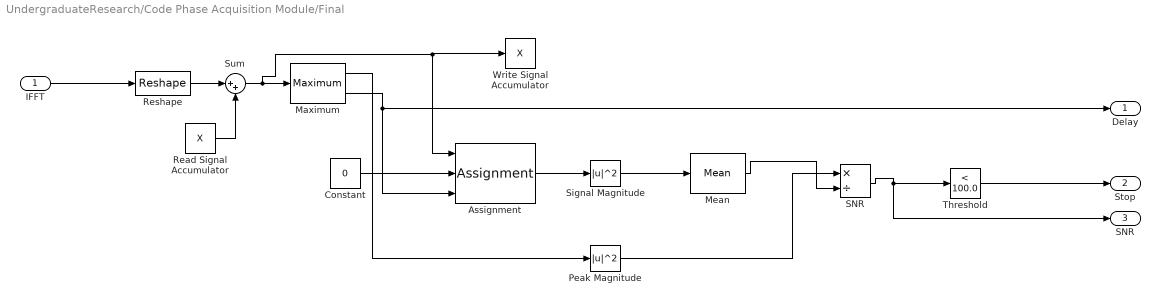
== system UndergraduateResearch/Code Phase Acquisition Module/Final ==
  IFFT : Inport
  " Read Signal Accumulator" : DataStoreRead  DataStoreName=X
  Assignment : Assignment  IndexOptions=Index vector (port)  Indices=1  OutputSizes=1
  Constant : Constant  Value=0
  Maximum : dspstat3/Maximum  fcn=Value and Index  reset=None  InputProcessing=Columns as channels (frame based)  indexBase=One  operateOver=Each column  Dimension=1  colComp=on  operation=maximum  roiEnable=off  roiType=Rectangles  roiPortion=Entire ROI  roiOutput=Individual statistics for each ROI  roiFlag=off  accumDataTypeStr=Inherit: Same as product output  accumLastDataTypeStr=Inherit: Same as product output  roundingMode=Floor  overflowMode=off
  Mean : dspstat3/Mean  run=off  reset_popup=None  InputProcessing=Columns as channels (frame based)  directionMode=Each column  dimension=1  treatSBRowAsCol=on  roiEnable=off  roiType=Rectangles  roiPortion=Entire ROI  roiOutput=Individual statistics for each ROI  roiFlag=off  outputDataTypeStr=Inherit: Same as accumulator  outputLastDataTypeStr=Inherit: Same as accumulator  outputMin=[]  outputMax=[]  roundingMode=Floor  overflowMode=off
  Peak Magnitude : Math  Operator=magnitude^2  SaturateOnIntegerOverflow=on
  Reshape : Reshape  OutputDimensions=[1023,40]
  SNR : Product  Inputs=*/
  Signal Magnitude : Math  Operator=magnitude^2  SaturateOnIntegerOverflow=on
  Sum : Sum  Inputs=|++
  Threshold : simulink/Logic and Bit Operations/Compare To Constant  relop=<  const=100.0  OutDataTypeStr=boolean
  Write Signal Accumulator : DataStoreWrite  DataStoreName=X
  Delay : Outport
  Stop : Outport  Port=2
  "SNR " : Outport  Port=3
  wires:
  Threshold/1 -> Stop/1
  Maximum/1 -> Peak Magnitude/1
  Maximum/2 -> Delay/1, Assignment/3
  Mean/1 -> SNR/2
  SNR/1 -> "SNR "/1, Threshold/1
  Sum/1 -> Assignment/1, Write Signal Accumulator/1, Maximum/1
  " Read Signal Accumulator"/1 -> Sum/2
  Assignment/1 -> Signal Magnitude/1
  Signal Magnitude/1 -> Mean/1
  Peak Magnitude/1 -> SNR/1
  Constant/1 -> Assignment/2
  Reshape/1 -> Sum/1
  IFFT/1 -> Reshape/1

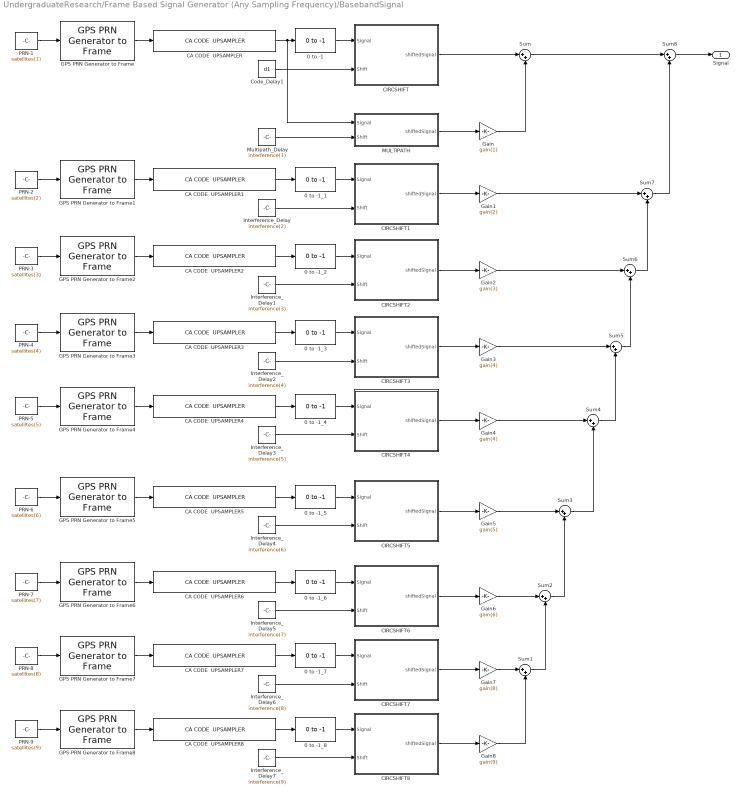
== system UndergraduateResearch/Frame Based Signal Generator (Any Sampling Frequency)/BasebandSignal ==
  " 0 to -1" : UndergraduateResearch/ 0 to -1
   0 to -1_{1..8} (8 alike) : UndergraduateResearch/ 0 to -1
  CA CODE  UPSAMPLER{,1..8} (9 alike) : UndergraduateResearch/CA CODE  UPSAMPLER  fs=fs
  CIRCSHIFT : MATLAB Function  TreatAsAtomicUnit=on  mask(CircularShift){}
      mask help: The block performs a circular shift of the Signal by the amount specified by Shift, the block is equivalent to the "circshift" function of MATLAB
  CIRCSHIFT1 : MATLAB Function  TreatAsAtomicUnit=on  mask(CircularShift){}
      mask help: The block performs a circular shift of the Signal by the amount specified by Shift, the block is equivalent to the "circshift" function of MATLAB
  CIRCSHIFT2 : MATLAB Function  TreatAsAtomicUnit=on  mask(CircularShift){}
      mask help: The block performs a circular shift of the Signal by the amount specified by Shift, the block is equivalent to the "circshift" function of MATLAB
  CIRCSHIFT3 : MATLAB Function  TreatAsAtomicUnit=on  mask(CircularShift){}
      mask help: The block performs a circular shift of the Signal by the amount specified by Shift, the block is equivalent to the "circshift" function of MATLAB
  CIRCSHIFT4 : MATLAB Function  TreatAsAtomicUnit=on  mask(CircularShift){}
      mask help: The block performs a circular shift of the Signal by the amount specified by Shift, the block is equivalent to the "circshift" function of MATLAB
  CIRCSHIFT5 : MATLAB Function  TreatAsAtomicUnit=on  mask(CircularShift){}
      mask help: The block performs a circular shift of the Signal by the amount specified by Shift, the block is equivalent to the "circshift" function of MATLAB
  CIRCSHIFT6 : MATLAB Function  TreatAsAtomicUnit=on  mask(CircularShift){}
      mask help: The block performs a circular shift of the Signal by the amount specified by Shift, the block is equivalent to the "circshift" function of MATLAB
  CIRCSHIFT7 : MATLAB Function  TreatAsAtomicUnit=on  mask(CircularShift){}
      mask help: The block performs a circular shift of the Signal by the amount specified by Shift, the block is equivalent to the "circshift" function of MATLAB
  CIRCSHIFT8 : MATLAB Function  TreatAsAtomicUnit=on  mask(CircularShift){}
      mask help: The block performs a circular shift of the Signal by the amount specified by Shift, the block is equivalent to the "circshift" function of MATLAB
  Code_Delay1 : Constant  Value=d1
  GPS PRN Generator to Frame{,1..8} (9 alike) : UndergraduateResearch/GPS PRN Generator to Frame
  Gain : Gain  Gain=gain(1)
  Gain1 : Gain  Gain=gain(2)
  Gain2 : Gain  Gain=gain(3)
  Gain3 : Gain  Gain=gain(4)
  Gain4 : Gain  Gain=gain(4)
  Gain5 : Gain  Gain=gain(5)
  Gain6 : Gain  Gain=gain(6)
  Gain7 : Gain  Gain=gain(8)
  Gain8 : Gain  Gain=gain(9)
  Interference_Delay : Constant  Value=interference(2)
  Interference_Delay1 : Constant  Value=interference(3)
  Interference_Delay2 : Constant  Value=interference(4)
  Interference_Delay3 : Constant  Value=interference(5)
  Interference_Delay4 : Constant  Value=interference(6)
  Interference_Delay5 : Constant  Value=interference(7)
  Interference_Delay6 : Constant  Value=interference(8)
  Interference_Delay7 : Constant  Value=interference(9)
  MULTIPATH : MATLAB Function  TreatAsAtomicUnit=on  mask(CircularShift){}
      mask help: The block performs a circular shift of the Signal by the amount specified by Shift, the block is equivalent to the "circshift" function of MATLAB
  Multipath_Delay : Constant  Value=interference(1)
  PRN-1 : Constant  Value=satellites(1)
  PRN-2 : Constant  Value=satellites(2)
  PRN-3 : Constant  Value=satellites(3)
  PRN-4 : Constant  Value=satellites(4)
  PRN-5 : Constant  Value=satellites(5)
  PRN-6 : Constant  Value=satellites(6)
  PRN-7 : Constant  Value=satellites(7)
  PRN-8 : Constant  Value=satellites(8)
  PRN-9 : Constant  Value=satellites(9)
  Sum{,1..8} (9 alike) : Sum  Inputs=|++
  Signal : Outport
  wires:
  CA CODE  UPSAMPLER2/1 -> " 0 to -1_2"/1
  Interference_Delay3/1 -> CIRCSHIFT4/2(Shift)
  CA CODE  UPSAMPLER/1 -> " 0 to -1"/1, MULTIPATH/1(Signal)
  Interference_Delay6/1 -> CIRCSHIFT7/2(Shift)
  " 0 to -1_8"/1 -> CIRCSHIFT8/1(Signal)
  CIRCSHIFT1/1(shiftedSignal) -> Gain1/1
  Interference_Delay5/1 -> CIRCSHIFT6/2(Shift)
  CIRCSHIFT3/1(shiftedSignal) -> Gain3/1
  Interference_Delay/1 -> CIRCSHIFT1/2(Shift)
  Sum1/1 -> Sum2/2
  GPS PRN Generator to Frame/1 -> CA CODE  UPSAMPLER/1
  CIRCSHIFT4/1(shiftedSignal) -> Gain4/1
  GPS PRN Generator to Frame1/1 -> CA CODE  UPSAMPLER1/1
  PRN-8/1 -> GPS PRN Generator to Frame7/1
  CA CODE  UPSAMPLER5/1 -> " 0 to -1_5"/1
  Sum6/1 -> Sum7/2
  Gain1/1 -> Sum7/1
  PRN-1/1 -> GPS PRN Generator to Frame/1
  Gain7/1 -> Sum1/1
  GPS PRN Generator to Frame3/1 -> CA CODE  UPSAMPLER3/1
  Sum3/1 -> Sum4/2
  PRN-3/1 -> GPS PRN Generator to Frame2/1
  PRN-6/1 -> GPS PRN Generator to Frame5/1
  Sum5/1 -> Sum6/2
  GPS PRN Generator to Frame4/1 -> CA CODE  UPSAMPLER4/1
  " 0 to -1_2"/1 -> CIRCSHIFT2/1(Signal)
  " 0 to -1_7"/1 -> CIRCSHIFT7/1(Signal)
  Code_Delay1/1 -> CIRCSHIFT/2(Shift)
  PRN-7/1 -> GPS PRN Generator to Frame6/1
  Gain4/1 -> Sum4/1
  CIRCSHIFT8/1(shiftedSignal) -> Gain8/1
  Interference_Delay1/1 -> CIRCSHIFT2/2(Shift)
  Gain8/1 -> Sum1/2
  Sum8/1 -> Signal/1
  CA CODE  UPSAMPLER6/1 -> " 0 to -1_6"/1
  " 0 to -1_1"/1 -> CIRCSHIFT1/1(Signal)
  Gain5/1 -> Sum3/1
  PRN-5/1 -> GPS PRN Generator to Frame4/1
  Interference_Delay4/1 -> CIRCSHIFT5/2(Shift)
  CIRCSHIFT5/1(shiftedSignal) -> Gain5/1
  GPS PRN Generator to Frame5/1 -> CA CODE  UPSAMPLER5/1
  CIRCSHIFT7/1(shiftedSignal) -> Gain7/1
  CA CODE  UPSAMPLER7/1 -> " 0 to -1_7"/1
  Interference_Delay7/1 -> CIRCSHIFT8/2(Shift)
  Gain6/1 -> Sum2/1
  Multipath_Delay/1 -> MULTIPATH/2(Shift)
  Sum7/1 -> Sum8/2
  " 0 to -1_5"/1 -> CIRCSHIFT5/1(Signal)
  Sum2/1 -> Sum3/2
  GPS PRN Generator to Frame8/1 -> CA CODE  UPSAMPLER8/1
  CIRCSHIFT6/1(shiftedSignal) -> Gain6/1
  " 0 to -1_6"/1 -> CIRCSHIFT6/1(Signal)
  Gain3/1 -> Sum5/1
  CIRCSHIFT/1(shiftedSignal) -> Sum/1
  GPS PRN Generator to Frame6/1 -> CA CODE  UPSAMPLER6/1
  CA CODE  UPSAMPLER8/1 -> " 0 to -1_8"/1
  Interference_Delay2/1 -> CIRCSHIFT3/2(Shift)
  GPS PRN Generator to Frame7/1 -> CA CODE  UPSAMPLER7/1
  Gain2/1 -> Sum6/1
  " 0 to -1"/1 -> CIRCSHIFT/1(Signal)
  PRN-4/1 -> GPS PRN Generator to Frame3/1
  GPS PRN Generator to Frame2/1 -> CA CODE  UPSAMPLER2/1
  " 0 to -1_4"/1 -> CIRCSHIFT4/1(Signal)
  " 0 to -1_3"/1 -> CIRCSHIFT3/1(Signal)
  CA CODE  UPSAMPLER3/1 -> " 0 to -1_3"/1
  Gain/1 -> Sum/2
  PRN-9/1 -> GPS PRN Generator to Frame8/1
  CA CODE  UPSAMPLER4/1 -> " 0 to -1_4"/1
  Sum4/1 -> Sum5/2
  PRN-2/1 -> GPS PRN Generator to Frame1/1
  MULTIPATH/1(shiftedSignal) -> Gain/1
  CA CODE  UPSAMPLER1/1 -> " 0 to -1_1"/1
  Sum/1 -> Sum8/1
  CIRCSHIFT2/1(shiftedSignal) -> Gain2/1

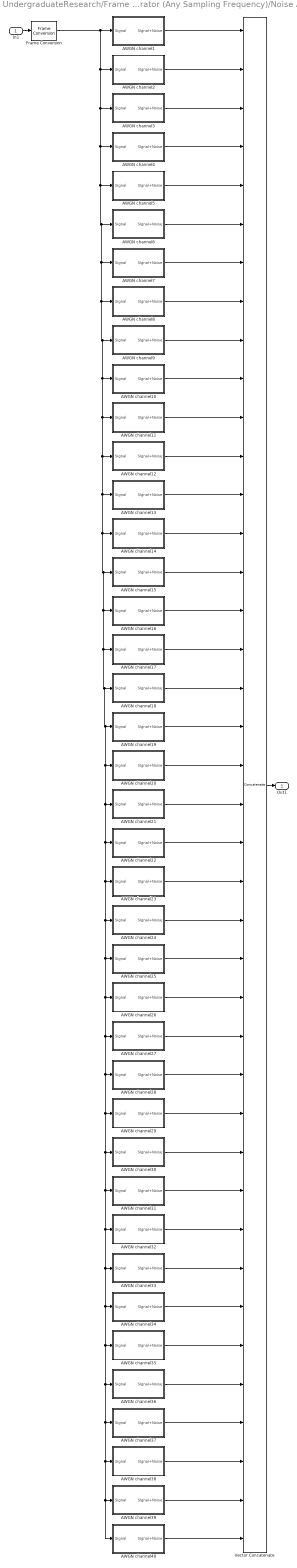
== system UndergraduateResearch/Frame Based Signal Generator (Any Sampling Frequency)/Noise Addition ==
  In1 : Inport
  AWGN channel1 : Subsystem
  AWGN channel10 : Subsystem
  AWGN channel11 : Subsystem
  AWGN channel12 : Subsystem
  AWGN channel13 : Subsystem
  AWGN channel14 : Subsystem
  AWGN channel15 : Subsystem
  AWGN channel16 : Subsystem
  AWGN channel17 : Subsystem
  AWGN channel18 : Subsystem
  AWGN channel19 : Subsystem
  AWGN channel2 : Subsystem
  AWGN channel20 : Subsystem
  AWGN channel21 : Subsystem
  AWGN channel22 : Subsystem
  AWGN channel23 : Subsystem
  AWGN channel24 : Subsystem
  AWGN channel25 : Subsystem
  AWGN channel26 : Subsystem
  AWGN channel27 : Subsystem
  AWGN channel28 : Subsystem
  AWGN channel29 : Subsystem
  AWGN channel3 : Subsystem
  AWGN channel30 : Subsystem
  AWGN channel31 : Subsystem
  AWGN channel32 : Subsystem
  AWGN channel33 : Subsystem
  AWGN channel34 : Subsystem
  AWGN channel35 : Subsystem
  AWGN channel36 : Subsystem
  AWGN channel37 : Subsystem
  AWGN channel38 : Subsystem
  AWGN channel39 : Subsystem
  AWGN channel4 : Subsystem
  AWGN channel40 : Subsystem
  AWGN channel5 : Subsystem
  AWGN channel6 : Subsystem
  AWGN channel7 : Subsystem
  AWGN channel8 : Subsystem
  AWGN channel9 : Subsystem
  Frame Conversion : FrameConversion  OutFrame=Sample-based
  Vector Concatenate : Concatenate  NumInputs=40
  Out1 : Outport
  wires:
  Vector Concatenate/1 -> Out1/1
  AWGN channel35/1(SIgnal+Noise) -> Vector Concatenate/35
  AWGN channel5/1(SIgnal+Noise) -> Vector Concatenate/5
  AWGN channel2/1(SIgnal+Noise) -> Vector Concatenate/2
  AWGN channel11/1(SIgnal+Noise) -> Vector Concatenate/11
  AWGN channel16/1(SIgnal+Noise) -> Vector Concatenate/16
  AWGN channel33/1(SIgnal+Noise) -> Vector Concatenate/33
  AWGN channel21/1(SIgnal+Noise) -> Vector Concatenate/21
  AWGN channel23/1(SIgnal+Noise) -> Vector Concatenate/23
  AWGN channel22/1(SIgnal+Noise) -> Vector Concatenate/22
  AWGN channel28/1(SIgnal+Noise) -> Vector Concatenate/28
  AWGN channel27/1(SIgnal+Noise) -> Vector Concatenate/27
  AWGN channel26/1(SIgnal+Noise) -> Vector Concatenate/26
  AWGN channel34/1(SIgnal+Noise) -> Vector Concatenate/34
  AWGN channel29/1(SIgnal+Noise) -> Vector Concatenate/29
  AWGN channel31/1(SIgnal+Noise) -> Vector Concatenate/31
  AWGN channel30/1(SIgnal+Noise) -> Vector Concatenate/30
  AWGN channel32/1(SIgnal+Noise) -> Vector Concatenate/32
  AWGN channel15/1(SIgnal+Noise) -> Vector Concatenate/15
  AWGN channel13/1(SIgnal+Noise) -> Vector Concatenate/13
  AWGN channel17/1(SIgnal+Noise) -> Vector Concatenate/17
  AWGN channel18/1(SIgnal+Noise) -> Vector Concatenate/18
  AWGN channel19/1(SIgnal+Noise) -> Vector Concatenate/19
  AWGN channel24/1(SIgnal+Noise) -> Vector Concatenate/24
  AWGN channel20/1(SIgnal+Noise) -> Vector Concatenate/20
  AWGN channel12/1(SIgnal+Noise) -> Vector Concatenate/12
  AWGN channel6/1(SIgnal+Noise) -> Vector Concatenate/6
  AWGN channel1/1(SIgnal+Noise) -> Vector Concatenate/1
  AWGN channel3/1(SIgnal+Noise) -> Vector Concatenate/3
  AWGN channel36/1(SIgnal+Noise) -> Vector Concatenate/36
  In1/1 -> Frame Conversion/1
  AWGN channel9/1(SIgnal+Noise) -> Vector Concatenate/9
  AWGN channel39/1(SIgnal+Noise) -> Vector Concatenate/39
  AWGN channel10/1(SIgnal+Noise) -> Vector Concatenate/10
  AWGN channel37/1(SIgnal+Noise) -> Vector Concatenate/37
  AWGN channel38/1(SIgnal+Noise) -> Vector Concatenate/38
  AWGN channel40/1(SIgnal+Noise) -> Vector Concatenate/40
  AWGN channel14/1(SIgnal+Noise) -> Vector Concatenate/14
  AWGN channel4/1(SIgnal+Noise) -> Vector Concatenate/4
  Frame Conversion/1 -> AWGN channel5/1(Signal), AWGN channel22/1(Signal), AWGN channel23/1(Signal), AWGN channel24/1(Signal), AWGN channel25/1(Signal), AWGN channel26/1(Signal), AWGN channel28/1(Signal), AWGN channel29/1(Signal), AWGN channel30/1(Signal), AWGN channel31/1(Signal), AWGN channel32/1(Signal), AWGN channel33/1(Signal), AWGN channel35/1(Signal), AWGN channel36/1(Signal), AWGN channel37/1(Signal), AWGN channel38/1(Signal), AWGN channel39/1(Signal), AWGN channel40/1(Signal), AWGN channel34/1(Signal), AWGN channel27/1(Signal), AWGN channel21/1(Signal), AWGN channel20/1(Signal), AWGN channel19/1(Signal), AWGN channel18/1(Signal), AWGN channel17/1(Signal), AWGN channel16/1(Signal), AWGN channel15/1(Signal), AWGN channel14/1(Signal), AWGN channel13/1(Signal), AWGN channel12/1(Signal), AWGN channel11/1(Signal), AWGN channel10/1(Signal), AWGN channel9/1(Signal), AWGN channel8/1(Signal), AWGN channel7/1(Signal), AWGN channel6/1(Signal), AWGN channel4/1(Signal), AWGN channel3/1(Signal), AWGN channel2/1(Signal), AWGN channel1/1(Signal)
  AWGN channel25/1(SIgnal+Noise) -> Vector Concatenate/25
  AWGN channel8/1(SIgnal+Noise) -> Vector Concatenate/8
  AWGN channel7/1(SIgnal+Noise) -> Vector Concatenate/7

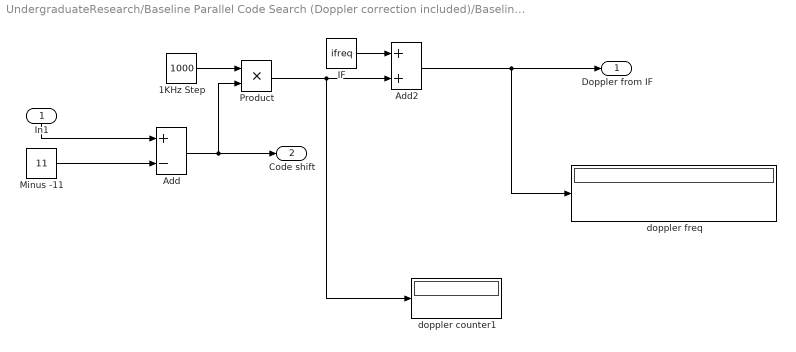
== system UndergraduateResearch/Baseline Parallel Code Search (Doppler correction included)/Baseline Code Phase Acquisition Module/Doppler Detector ==
  In1 : Inport
  1KHz Step : Constant  Value=1000
  Add : Sum  Inputs=+-
  Add2 : Sum
  IF : Constant  Value=ifreq
  Minus -11 : Constant  Value=11
  Product : Product
  doppler counter1 : Display
  doppler freq : Display
  Doppler from IF : Outport
  Code shift : Outport  Port=2
  wires:
  Add/1 -> Product/2, Code shift/1
  In1/1 -> Add/1
  Minus -11/1 -> Add/2
  IF/1 -> Add2/1
  Add2/1 -> Doppler from IF/1, doppler freq/1
  1KHz Step/1 -> Product/1
  Product/1 -> doppler counter1/1, Add2/2

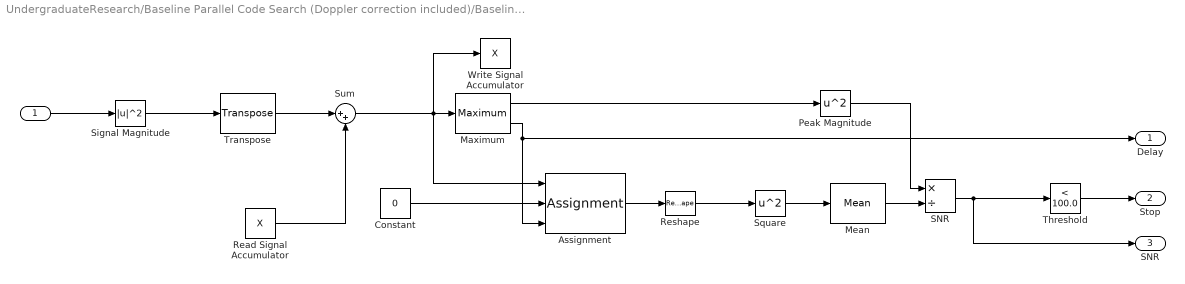
== system UndergraduateResearch/Baseline Parallel Code Search (Doppler correction included)/Baseline Code Phase Acquisition Module/Final ==
  " " : Inport
  " Read Signal Accumulator" : DataStoreRead  DataStoreName=X
  Assignment : Assignment  IndexOptions=Index vector (port)  Indices=1  OutputSizes=1
  Constant : Constant  Value=0
  Maximum : dspstat3/Maximum  fcn=Value and Index  reset=None  InputProcessing=Columns as channels (frame based)  indexBase=One  operateOver=Each column  Dimension=1  colComp=on  operation=maximum  roiEnable=off  roiType=Rectangles  roiPortion=Entire ROI  roiOutput=Individual statistics for each ROI  roiFlag=off  accumDataTypeStr=Inherit: Same as product output  accumLastDataTypeStr=Inherit: Same as product output  roundingMode=Floor  overflowMode=off
  Mean : dspstat3/Mean  run=off  reset_popup=None  InputProcessing=Columns as channels (frame based)  directionMode=Entire input  dimension=1  treatSBRowAsCol=on  roiEnable=off  roiType=Rectangles  roiPortion=Entire ROI  roiOutput=Individual statistics for each ROI  roiFlag=off  outputDataTypeStr=Inherit: Same as accumulator  outputLastDataTypeStr=Inherit: Same as accumulator  outputMin=[]  outputMax=[]  roundingMode=Floor  overflowMode=off
  Peak Magnitude : Math  Operator=square  SaturateOnIntegerOverflow=on
  Reshape : Reshape
  SNR : Product  Inputs=*/
  Signal Magnitude : Math  Operator=magnitude^2  SaturateOnIntegerOverflow=on
  Square : Math  Operator=square  SaturateOnIntegerOverflow=on
  Sum : Sum  Inputs=|++
  Threshold : simulink/Logic and Bit Operations/Compare To Constant  relop=<  const=100.0  OutDataTypeStr=boolean
  Transpose : dspmtrx3/Transpose  Hermitian=off  overflowFlag=off
  Write Signal Accumulator : DataStoreWrite  DataStoreName=X
  Delay : Outport
  Stop : Outport  Port=2
  "SNR " : Outport  Port=3
  wires:
  Maximum/2 -> Delay/1, Assignment/3
  Constant/1 -> Assignment/2
  Reshape/1 -> Square/1
  Assignment/1 -> Reshape/1
  Signal Magnitude/1 -> Transpose/1
  Transpose/1 -> Sum/1
  " "/1 -> Signal Magnitude/1
  " Read Signal Accumulator"/1 -> Sum/2
  Sum/1 -> Maximum/1, Write Signal Accumulator/1, Assignment/1
  Peak Magnitude/1 -> SNR/1
  Square/1 -> Mean/1
  SNR/1 -> Threshold/1, "SNR "/1
  Mean/1 -> SNR/2
  Maximum/1 -> Peak Magnitude/1
  Threshold/1 -> Stop/1

== system UndergraduateResearch/Frame Based Signal Generator (Any Sampling Frequency)/Noise Addition/AWGN channel1 ==
  Signal : Inport
  AWGN Channel : commchan3/AWGN Channel  InputProcessing=Columns as channels (frame based)  seed=10  noiseMode="Signal to noise ratio  (SNR)"  EbNodB=10  EsNodB=10  SNRdB=-20  bitsPerSym=1  Ps=1  Tsym=1  variance=1
  Frame Conversion : FrameConversion  OutFrame=Sample-based
  SIgnal+Noise : Outport
  wires:
  Signal/1 -> AWGN Channel/1
  AWGN Channel/1 -> Frame Conversion/1
  Frame Conversion/1 -> SIgnal+Noise/1

== system UndergraduateResearch/Frame Based Signal Generator (Any Sampling Frequency)/Noise Addition/AWGN channel10 ==
  Signal : Inport
  AWGN Channel : commchan3/AWGN Channel  InputProcessing=Columns as channels (frame based)  seed=10  noiseMode="Signal to noise ratio  (SNR)"  EbNodB=10  EsNodB=10  SNRdB=-20  bitsPerSym=1  Ps=1  Tsym=1  variance=1
  Frame Conversion : FrameConversion  OutFrame=Sample-based
  SIgnal+Noise : Outport
  wires:
  Signal/1 -> AWGN Channel/1
  AWGN Channel/1 -> Frame Conversion/1
  Frame Conversion/1 -> SIgnal+Noise/1

== system UndergraduateResearch/Frame Based Signal Generator (Any Sampling Frequency)/Noise Addition/AWGN channel11 ==
  Signal : Inport
  AWGN Channel : commchan3/AWGN Channel  InputProcessing=Columns as channels (frame based)  seed=11  noiseMode="Signal to noise ratio  (SNR)"  EbNodB=10  EsNodB=10  SNRdB=-20  bitsPerSym=1  Ps=1  Tsym=1  variance=1
  Frame Conversion : FrameConversion  OutFrame=Sample-based
  SIgnal+Noise : Outport
  wires:
  Signal/1 -> AWGN Channel/1
  AWGN Channel/1 -> Frame Conversion/1
  Frame Conversion/1 -> SIgnal+Noise/1

== system UndergraduateResearch/Frame Based Signal Generator (Any Sampling Frequency)/Noise Addition/AWGN channel12 ==
  Signal : Inport
  AWGN Channel : commchan3/AWGN Channel  InputProcessing=Columns as channels (frame based)  seed=12  noiseMode="Signal to noise ratio  (SNR)"  EbNodB=10  EsNodB=10  SNRdB=-20  bitsPerSym=1  Ps=1  Tsym=1  variance=1
  Frame Conversion : FrameConversion  OutFrame=Sample-based
  SIgnal+Noise : Outport
  wires:
  Signal/1 -> AWGN Channel/1
  AWGN Channel/1 -> Frame Conversion/1
  Frame Conversion/1 -> SIgnal+Noise/1

== system UndergraduateResearch/Frame Based Signal Generator (Any Sampling Frequency)/Noise Addition/AWGN channel13 ==
  Signal : Inport
  AWGN Channel : commchan3/AWGN Channel  InputProcessing=Columns as channels (frame based)  seed=13  noiseMode="Signal to noise ratio  (SNR)"  EbNodB=10  EsNodB=10  SNRdB=-20  bitsPerSym=1  Ps=1  Tsym=1  variance=1
  Frame Conversion : FrameConversion  OutFrame=Sample-based
  SIgnal+Noise : Outport
  wires:
  Signal/1 -> AWGN Channel/1
  AWGN Channel/1 -> Frame Conversion/1
  Frame Conversion/1 -> SIgnal+Noise/1

== system UndergraduateResearch/Frame Based Signal Generator (Any Sampling Frequency)/Noise Addition/AWGN channel14 ==
  Signal : Inport
  AWGN Channel : commchan3/AWGN Channel  InputProcessing=Columns as channels (frame based)  seed=14  noiseMode="Signal to noise ratio  (SNR)"  EbNodB=10  EsNodB=10  SNRdB=-20  bitsPerSym=1  Ps=1  Tsym=1  variance=1
  Frame Conversion : FrameConversion  OutFrame=Sample-based
  SIgnal+Noise : Outport
  wires:
  Signal/1 -> AWGN Channel/1
  AWGN Channel/1 -> Frame Conversion/1
  Frame Conversion/1 -> SIgnal+Noise/1

== system UndergraduateResearch/Frame Based Signal Generator (Any Sampling Frequency)/Noise Addition/AWGN channel15 ==
  Signal : Inport
  AWGN Channel : commchan3/AWGN Channel  InputProcessing=Columns as channels (frame based)  seed=15  noiseMode="Signal to noise ratio  (SNR)"  EbNodB=10  EsNodB=10  SNRdB=-20  bitsPerSym=1  Ps=1  Tsym=1  variance=1
  Frame Conversion : FrameConversion  OutFrame=Sample-based
  SIgnal+Noise : Outport
  wires:
  Signal/1 -> AWGN Channel/1
  AWGN Channel/1 -> Frame Conversion/1
  Frame Conversion/1 -> SIgnal+Noise/1
